simulink model "TV_2018_HIL"  (R2016a)
settings: Solver=FixedStepAuto  StartTime=0.0  StopTime=inf  FixedStep=0.001  RelTol=1e-3
PreLoadFcn:
  | TV_2017_parameters
values from neighbouring files (symbols this model uses):
  battery_voltage = single(530)    [HIL_parameters.m]    (also in HIL_parameters_2018.m; TV_2017_parameters.m; TV_2017_parameters_VD.m)
  car_params = Simulink_Car_params    [HIL_parameters.m]    (also in HIL_parameters_2018.m; TV_2017_parameters.m; TV_2017_parameters_VD.m)
  i_Diff = 16    [HIL_parameters.m]    (also in HIL_parameters_2018.m; TV_2017_parameters.m)
  Kp = 1    [HIL_parameters.m]    (also in HIL_parameters_2018.m; TV_2017_parameters.m; TV_2017_parameters_VD.m)
  motor_data = struct    [HIL_parameters.m]    (also in HIL_parameters_2018.m; TV_2017_parameters.m)
  powerLimitControl = Simulink_el    [HIL_parameters.m]    (also in HIL_parameters_2018.m; TV_2017_parameters.m; TV_2017_parameters_VD.m)
  settings = Simulink_Settings    [HIL_parameters.m]    (also in HIL_parameters_2018.m; TV_2017_parameters.m; TV_2017_parameters_VD.m)
  SpdC_BCC = 0    [HIL_parameters.m]    (also in HIL_parameters_2018.m; TV_2017_parameters.m; TV_2017_parameters_VD.m)
  Speed_Neg_sat = -21    [HIL_parameters.m]    (also in HIL_parameters_2018.m; TV_2017_parameters.m; TV_2017_parameters_VD.m)
  Speed_Pos_sat = 21    [HIL_parameters.m]    (also in HIL_parameters_2018.m; TV_2017_parameters.m; TV_2017_parameters_VD.m)
  SteeringAngleFL = [-23.80 -22.65 -21.50 -20.34 -19.18 -18.03 -16.86 -15.70 -14.53 -13.35 -12.18 -10.99 -9.80 -8.61 -7.40 -6.19 -4.97 -3.75 -2.51 -1.26 0 1.27 2.56 3.85 5.17 6.50 7.84 9.21 10.59 12.00 13.42 14.88 16.36 17.87 19.41 20.99 22.61 24.26 25.97 27.73 29.54]    [CarSetupAnalysis2018.m]    (also in HIL_parameters_2018.m; TV_2017_parameters.m; TV_2017_parameters_VD.m = [-24.129 -22.950 -21.772 -20.593 -19.413 -18.232 -17.050 -15)
  SteeringAngleFR = [-29.54 -27.73 -25.97 -24.26 -22.61 -20.99 -19.41 -17.87 -16.36 -14.88 -13.42 -12.00 -10.59 -9.21 -7.84 -6.50 -5.17 -3.85 -2.56 -1.27 0 1.26 2.51 3.75 4.97 6.19 7.40 8.61 9.80 10.99 12.18 13.35 14.53 15.70 16.86 18.03 19.18 20.34 21.50 22.65 23.80]    [CarSetupAnalysis2018.m]    (also in HIL_parameters_2018.m; TV_2017_parameters.m; TV_2017_parameters_VD.m = [-29.3050 -27.5340 -25.8140 -24.1410 -22.5110 -20.9180 -19.3)
  SteeringWhAngle = [-105 -99.75 -94.5 -89.25 -84 -78.75 -73.5 -68.25 -63 -57.75 -52.5 -47.25 -42 -36.75 -31.5 -26.25 -21.0 -15.75 -10.5 -5.25 0.0 5.25 10.50 15.75 21.00 26.25 31.50 36.75 42.00 47.25 52.50 57.75  63.00 68.25 73.50 78.75 84.00 89.25 94.50 99.75 105.00]    [TV_2017_parameters_VD.m]
  Tn_n = 0    [HIL_parameters.m]    (also in HIL_parameters_2018.m; TV_2017_parameters.m; TV_2017_parameters_VD.m)
  tractionControl = Simulink_tc    [HIL_parameters.m]    (also in HIL_parameters_2018.m; IterativeTractionControlTuning.m; TV_2017_parameters.m; TV_2017_parameters_VD.m)
  yawMomentGenerator = struct    [HIL_parameters.m]    (also in HIL_parameters_2018.m = Simulink_yawRate2; TV_2017_parameters.m = Simulink_yawRate2)
  yawRateControl = Simulink_yawRate    [HIL_parameters.m]    (also in HIL_parameters_2018.m; TV_2017_parameters.m; TV_2017_parameters_VD.m)
undefined symbols (not defined in the file or in its folder): canChannel, DiscIntNeverNeededParam, magnitude, speedEstimation, TC_Decr_Gas, TC_Derivative, TC_Incr_Gas, TC_On, TC_Relay_Off, TC_Relay_On
libraries: CarMaker4SL x366, simulink_extras x63, canmsglib x55, canlib x41, simulink x37, dspfdesign x2, sldrtlib x1
(part 4 of 15)

== system TV_2018_HIL/CarMaker/Send sensor data and driver input to microcontroller /If Action Subsystem1 ==
  Action Port : ActionPort
  CAN Pack24 : canmsglib/CAN Pack  MsgList=(none)  MsgName=CAN Msg  MsgIDType=Standard (11-bit identifier)  MsgIdentifier=DRIVE_ENABLE  MsgLength=0  NSignals=0  StartBits=0  SignalSizes=0  ByteOrders=0  DataTypes=0  MultiplexTypes=0  MultiplexValues=0  Factors=0  Offsets=0  Minimums=0  Maximums=0  Remote=off
      settings: DataFormat=manually specified signals
  CAN Transmit24 : canlib/CAN Transmit  BlockHandle=3115.0001  DeviceMenu=(none)  Device=PEAK-System PCAN-PCI Express (PCAN_PCIBUS1)  ObjConstructor=canChannel('PEAK-System', 'PCAN_PCIBUS1')  EnablePeriodicTransmit=off  MessagePeriod=1.000

== system TV_2018_HIL/CarMaker/Send sensor data and driver input to microcontroller /If Action Subsystem2 ==
  Action Port : ActionPort  ActionType=case
  CAN Pack23 : canmsglib/CAN Pack  MsgList=(none)  MsgName=CAN Msg  MsgIDType=Standard (11-bit identifier)  MsgIdentifier=RESET_INVERTER  MsgLength=0  NSignals=0  StartBits=0  SignalSizes=0  ByteOrders=0  DataTypes=0  MultiplexTypes=0  MultiplexValues=0  Factors=0  Offsets=0  Minimums=0  Maximums=0  Remote=off
      settings: DataFormat=manually specified signals
  CAN Transmit23 : canlib/CAN Transmit  BlockHandle=3119.0001  DeviceMenu=(none)  Device=PEAK-System PCAN-PCI Express (PCAN_PCIBUS1)  ObjConstructor=canChannel('PEAK-System', 'PCAN_PCIBUS1')  EnablePeriodicTransmit=off  MessagePeriod=1.000
  wires:
  CAN Pack23/1 -> CAN Transmit23/1

== system TV_2018_HIL/CarMaker/Send sensor data and driver input to microcontroller /Push Button ==

== system TV_2018_HIL/CarMaker/Send sensor data and driver input to microcontroller /Push Button1 ==

== system TV_2018_HIL/CarMaker/Send sensor data and driver input to microcontroller /Push Button2 ==

== system TV_2018_HIL/CarMaker/Send sensor data and driver input to microcontroller /Trash ==
  In1 : Inport
  In2 : Inport  Port=2
  In3 : Inport  Port=3
  In4 : Inport  Port=4
  In5 : Inport  Port=5
  In6 : Inport  Port=6
  In7 : Inport  Port=7
  In8 : Inport  Port=8
  In9 : Inport  Port=9
  In10 : Inport  Port=10
  In11 : Inport  Port=11
  In12 : Inport  Port=12
  In13 : Inport  Port=13
  In14 : Inport  Port=14
  In15 : Inport  Port=15
  In16 : Inport  Port=16
  In17 : Inport  Port=17
  In18 : Inport  Port=18
  CAN Pack : canmsglib/CAN Pack  Commented=on  MsgList=(none)  MsgName=CAN Msg  MsgIDType=Standard (11-bit identifier)  MsgIdentifier=ACD_DAMPER_FL_ID  MsgLength=2  SignalInfo=FL$0$16$1$1$1$0$1$0$-Inf$Inf$#  NSignals=1  StartBits=str2num('[int32(0)]')  SignalSizes=str2num('[int32(16)]')  ByteOrders=str2num('[int32(1)]')  DataTypes=str2num('[int32(1)]')  MultiplexTypes=str2num('[int32(1)]')  MultiplexValues=str2num('[double(0)]')  Factors=str2num('[double(1)]')  Offsets=str2num('[double(0)]')  Minimums=str2num('[double(-Inf)]')  Maximums=str2num('[double(Inf)]')  Remote=off
      settings: DataFormat=manually specified signals
  CAN Pack1 : canmsglib/CAN Pack  Commented=on  MsgList=(none)  MsgName=CAN Msg  MsgIDType=Standard (11-bit identifier)  MsgIdentifier=ACD_DAMPER_FR_ID  MsgLength=8  NSignals=0  StartBits=0  SignalSizes=0  ByteOrders=0  DataTypes=0  MultiplexTypes=0  MultiplexValues=0  Factors=0  Offsets=0  Minimums=0  Maximums=0  Remote=off
      settings: DataFormat=manually specified signals
  CAN Pack12 : canmsglib/CAN Pack  Commented=on  MsgList=(none)  MsgName=RPM  MsgIDType=Standard (11-bit identifier)  MsgIdentifier=502  MsgLength=8  SignalInfo=RPM_FL$0$16$1$1$1$0$1$0$-Inf$Inf$#RPM_FR$16$16$1$1$1$0$1$0$-Inf$Inf$#RPM_RL$32$16$1$1$1$0$1$0$-Inf$Inf$#RPM_RR$48$16$1$1$1$0$1$0$-Inf$Inf$#  NSignals=4  StartBits=str2num('[int32(0);int32(16);int32(32);int32(48)]')  SignalSizes=str2num('[int32(16);int32(16);int32(16);int32(16)]')  ByteOrders=str2num('[int32(1);int32(1);int32(1);int32(1)]')  DataTypes=str2num('[int32(1);int32(1);int32(1);int32(1)]')  MultiplexTypes=str2num('[int32(1);int32(1);int32(1);int32(1)]')  MultiplexValues=str2num('[double(0);double(0);double(0);double(0)]')  Factors=str2num('[double(1);double(1);double(1);double(1)]')  Offsets=str2num('[double(0);double(0);double(0);double(0)]')  Minimums=str2num('[double(-Inf);double(-Inf);double(-Inf);double(-Inf)]')  Maximums=str2num('[double(Inf);double(Inf);double(Inf);double(Inf)]')  Remote=off
      settings: DataFormat=manually specified signals
  CAN Pack2 : canmsglib/CAN Pack  Commented=on  MsgList=(none)  MsgName=CAN Msg  MsgIDType=Standard (11-bit identifier)  MsgIdentifier=ACD_DAMPER_RL_ID  MsgLength=8  NSignals=0  StartBits=0  SignalSizes=0  ByteOrders=0  DataTypes=0  MultiplexTypes=0  MultiplexValues=0  Factors=0  Offsets=0  Minimums=0  Maximums=0  Remote=off
      settings: DataFormat=manually specified signals
  CAN Pack20 : canmsglib/CAN Pack  Commented=on  MsgList=(none)  MsgName=Fz  MsgIDType=Standard (11-bit identifier)  MsgIdentifier=500  MsgLength=8  SignalInfo=Fz_FL$0$16$1$2$1$0$1$0$-Inf$Inf$#Fz_FR$16$16$1$2$1$0$1$0$-Inf$Inf$#Fz_RL$32$16$1$2$1$0$1$0$-Inf$Inf$#Fz_RR$48$16$1$2$1$0$1$0$-Inf$Inf$#  NSignals=4  StartBits=str2num('[int32(0);int32(16);int32(32);int32(48)]')  SignalSizes=str2num('[int32(16);int32(16);int32(16);int32(16)]')  ByteOrders=str2num('[int32(1);int32(1);int32(1);int32(1)]')  DataTypes=str2num('[int32(2);int32(2);int32(2);int32(2)]')  MultiplexTypes=str2num('[int32(1);int32(1);int32(1);int32(1)]')  MultiplexValues=str2num('[double(0);double(0);double(0);double(0)]')  Factors=str2num('[double(1);double(1);double(1);double(1)]')  Offsets=str2num('[double(0);double(0);double(0);double(0)]')  Minimums=str2num('[double(-Inf);double(-Inf);double(-Inf);double(-Inf)]')  Maximums=str2num('[double(Inf);double(Inf);double(Inf);double(Inf)]')  Remote=off
      settings: DataFormat=manually specified signals
  CAN Pack3 : canmsglib/CAN Pack  Commented=on  MsgList=(none)  MsgName=CAN Msg  MsgIDType=Standard (11-bit identifier)  MsgIdentifier=ACD_DAMPER_RR_ID  MsgLength=8  NSignals=0  StartBits=0  SignalSizes=0  ByteOrders=0  DataTypes=0  MultiplexTypes=0  MultiplexValues=0  Factors=0  Offsets=0  Minimums=0  Maximums=0  Remote=off
      settings: DataFormat=manually specified signals
  CAN Pack6 : canmsglib/CAN Pack  Commented=on  MsgList=(none)  MsgName=Senors  MsgIDType=Standard (11-bit identifier)  MsgIdentifier=501  MsgLength=8  SignalInfo=gas$0$8$1$2$1$0$1$0$-Inf$Inf$#kers$8$8$1$2$1$0$1$0$-Inf$Inf$#steering$16$16$1$1$1$0$1$0$-Inf$Inf$#vx$32$16$1$1$1$0$1$0$-Inf$Inf$#yawrate$48$16$1$1$1$0$1$0$-Inf$Inf$#  NSignals=5  StartBits=str2num('[int32(0);int32(8);int32(16);int32(32);int32(48)]')  SignalSizes=str2num('[int32(8);int32(8);int32(16);int32(16);int32(16)]')  ByteOrders=str2num('[int32(1);int32(1);int32(1);int32(1);int32(1)]')  DataTypes=str2num('[int32(2);int32(2);int32(1);int32(1);int32(1)]')  MultiplexTypes=str2num('[int32(1);int32(1);int32(1);int32(1);int32(1)]')  MultiplexValues=str2num('[double(0);double(0);double(0);double(0);double(0)]')  Factors=str2num('[double(1);double(1);double(1);double(1);double(1)]')  Offsets=str2num('[double(0);double(0);double(0);double(0);double(0)]')  Minimums=str2num('[double(-Inf);double(-Inf);double(-Inf);double(-Inf);double(-Inf)]')  Maximums=str2num('[double(Inf);double(Inf);double(Inf);double(Inf);double(Inf)]')  Remote=off
      settings: DataFormat=manually specified signals
  CAN Pack8 : canmsglib/CAN Pack  Commented=on  MsgList=(none)  MsgName=CAN Msg  MsgIDType=Standard (11-bit identifier)  MsgIdentifier=2  MsgLength=8  SignalInfo=Signal1$0$8$1$1$1$0$1$0$-Inf$Inf$#  NSignals=1  StartBits=str2num('[int32(0)]')  SignalSizes=str2num('[int32(8)]')  ByteOrders=str2num('[int32(1)]')  DataTypes=str2num('[int32(1)]')  MultiplexTypes=str2num('[int32(1)]')  MultiplexValues=str2num('[double(0)]')  Factors=str2num('[double(1)]')  Offsets=str2num('[double(0)]')  Minimums=str2num('[double(-Inf)]')  Maximums=str2num('[double(Inf)]')  Remote=off
      settings: DataFormat=manually specified signals
  CAN Transmit : canlib/CAN Transmit  Commented=on  BlockHandle=19242.0006  DeviceMenu=Kvaser Virtual 1 (Channel 1)  Device=PEAK-System PCAN-PCI Express (PCAN_PCIBUS1)  ObjConstructor=CANTRANCONSTRUCTOR  EnablePeriodicTransmit=off  MessagePeriod=1.000
  CAN Transmit1 : canlib/CAN Transmit  Commented=on  BlockHandle=19243.0006  DeviceMenu=Kvaser Virtual 1 (Channel 1)  Device=PEAK-System PCAN-USB (PCAN_USBBUS1)  ObjConstructor=canChannel('PEAK-System', 'PCAN_USBBUS1')  EnablePeriodicTransmit=on  MessagePeriod=0.01
  CAN Transmit15 : canlib/CAN Transmit  Commented=on  BlockHandle=19244.0006  DeviceMenu=Kvaser Virtual 1 (Channel 1)  Device=PEAK-System PCAN-USB (PCAN_USBBUS1)  ObjConstructor=canChannel('PEAK-System', 'PCAN_USBBUS1')  EnablePeriodicTransmit=on  MessagePeriod=0.01
  CAN Transmit19 : canlib/CAN Transmit  Commented=on  BlockHandle=19245.0006  DeviceMenu=Kvaser Virtual 1 (Channel 1)  Device=PEAK-System PCAN-USB (PCAN_USBBUS1)  ObjConstructor=canChannel('PEAK-System', 'PCAN_USBBUS1')  EnablePeriodicTransmit=on  MessagePeriod=0.01
  CAN Transmit2 : canlib/CAN Transmit  Commented=on  BlockHandle=19246.0006  DeviceMenu=Kvaser Virtual 1 (Channel 1)  Device=PEAK-System PCAN-PCI Express (PCAN_PCIBUS1)  ObjConstructor=CANTRANCONSTRUCTOR  EnablePeriodicTransmit=off  MessagePeriod=1.000
  CAN Transmit3 : canlib/CAN Transmit  Commented=on  BlockHandle=19247.0006  DeviceMenu=Kvaser Virtual 1 (Channel 1)  Device=PEAK-System PCAN-PCI Express (PCAN_PCIBUS1)  ObjConstructor=CANTRANCONSTRUCTOR  EnablePeriodicTransmit=off  MessagePeriod=1.000
  CAN Transmit4 : canlib/CAN Transmit  Commented=on  BlockHandle=19248.0006  DeviceMenu=Kvaser Virtual 1 (Channel 1)  Device=PEAK-System PCAN-PCI Express (PCAN_PCIBUS1)  ObjConstructor=CANTRANCONSTRUCTOR  EnablePeriodicTransmit=off  MessagePeriod=1.000
  CAN Transmit8 : canlib/CAN Transmit  Commented=on  BlockHandle=19249.0006  DeviceMenu=Kvaser Virtual 1 (Channel 1)  Device=PEAK-System PCAN-PCI Express (PCAN_PCIBUS1)  ObjConstructor=canChannel('PEAK-System', 'PCAN_PCIBUS1')  EnablePeriodicTransmit=off  MessagePeriod=1.000
  Constant5 : Constant  Commented=on
  Constant6 : Constant  Commented=on
  Scope11 : Scope  Commented=on
  Out1 : Outport
  wires:
  CAN Pack8/1 -> CAN Transmit8/1
  In9/1 -> CAN Pack6/2
  In8/1 -> CAN Pack6/1
  In10/1 -> CAN Pack6/3
  In18/1 -> Scope11/1
  In3/1 -> CAN Pack3/1
  In15/1 -> CAN Transmit15/1
  CAN Pack12/1 -> Out1/1
  In17/1 -> CAN Pack12/4
  In4/1 -> CAN Pack20/1
  In5/1 -> CAN Pack20/2
  In14/1 -> CAN Pack12/2
  In7/1 -> CAN Pack20/4
  In12/1 -> CAN Pack6/5
  In2/1 -> CAN Pack2/1
  In13/1 -> CAN Pack12/1
  In16/1 -> CAN Pack12/3
  In11/1 -> CAN Pack6/4
  In1/1 -> CAN Pack1/1
  In6/1 -> CAN Pack20/3
  CAN Pack6/1 -> CAN Transmit1/1
  CAN Pack3/1 -> CAN Transmit4/1
  CAN Pack/1 -> CAN Transmit/1
  Constant5/1 -> CAN Pack/1
  CAN Pack1/1 -> CAN Transmit2/1
  CAN Pack20/1 -> CAN Transmit19/1
  CAN Pack2/1 -> CAN Transmit3/1
  Constant6/1 -> CAN Pack8/1

== system TV_2018_HIL/CarMaker/Send sensor data and driver input to microcontroller /force2 0.1mmDamperFront ==
  In1 : Inport
  Constant2 : Constant  Value=800
  Gain : Gain  Gain=1/car_params.spring_constant_front
  Sum : Sum  Inputs=|++
  sensor scale : Gain  Gain=1/0.1
  Out1 : Outport
  wires:
  Constant2/1 -> Sum/2
  In1/1 -> Sum/1
  Sum/1 -> Gain/1
  Gain/1 -> sensor scale/1
  sensor scale/1 -> Out1/1

== system TV_2018_HIL/CarMaker/Send sensor data and driver input to microcontroller /force2mmDamperFront1 ==
  In1 : Inport
  Constant2 : Constant  Value=800
  Gain1 : Gain  Gain=1/car_params.spring_constant_front
  Sum : Sum  Inputs=|++
  sensor scale : Gain  Gain=1/0.1
  Out1 : Outport
  wires:
  Constant2/1 -> Sum/2
  In1/1 -> Sum/1
  Sum/1 -> Gain1/1
  Gain1/1 -> sensor scale/1
  sensor scale/1 -> Out1/1

== system TV_2018_HIL/CarMaker/Send sensor data and driver input to microcontroller /force2mmDamperRear ==
  In1 : Inport
  Constant2 : Constant  Value=1600
  Gain : Gain  Gain=1/car_params.spring_constant_rear
  Sum : Sum  Inputs=|++
  sensor scale : Gain  Gain=1/0.1
  Out1 : Outport
  wires:
  Constant2/1 -> Sum/2
  In1/1 -> Sum/1
  Sum/1 -> Gain/1
  Gain/1 -> sensor scale/1
  sensor scale/1 -> Out1/1

== system TV_2018_HIL/CarMaker/Send sensor data and driver input to microcontroller /force2mmDamperRear1 ==
  In1 : Inport
  Constant2 : Constant  Value=1600
  Gain : Gain  Gain=1/car_params.spring_constant_rear
  Sum : Sum  Inputs=|++
  sensor scale : Gain  Gain=1/0.1
  Out1 : Outport
  wires:
  Constant2/1 -> Sum/2
  In1/1 -> Sum/1
  Sum/1 -> Gain/1
  Gain/1 -> sensor scale/1
  sensor scale/1 -> Out1/1

== system TV_2018_HIL/CarMaker/Subsystem/Control Output to CarMaker model  ==
  "Ti_pos " : Inport
  Ti_neg : Inport  Port=2
  wi_ref : Inport  Port=3
  Bus Selector : BusSelector  OutputSignals=FL,FR,RL,RR
  Bus Selector1 : BusSelector  OutputSignals=FL,FR,RL,RR
  Bus Selector2 : BusSelector  OutputSignals=FL,FR,RL,RR
  Data Type Conversion{,1..11} (12 alike) : DataTypeConversion  OutDataTypeStr=double
  Gain{,1..7} (8 alike) : Gain  Gain=car_params.Mn
  Scope4 : Scope
  Ti_To_CarMaker : Scope  NumInputPorts=4
  Write CM Dict : CarMaker4SL/Write CM Dict  xname=T_req_RR  xsync=off
  Write CM Dict1 : CarMaker4SL/Write CM Dict  xname=T_req_RL  xsync=off
  Write CM Dict10 : CarMaker4SL/Write CM Dict  xname=Tlim_pos_RL  xsync=off
  Write CM Dict11 : CarMaker4SL/Write CM Dict  xname=Tlim_pos_RR  xsync=off
  Write CM Dict16 : CarMaker4SL/Write CM Dict  xname=Tlim_neg_FL  xsync=off
  Write CM Dict17 : CarMaker4SL/Write CM Dict  xname=Tlim_neg_FR  xsync=off
  Write CM Dict18 : CarMaker4SL/Write CM Dict  xname=Tlim_neg_RL  xsync=off
  Write CM Dict19 : CarMaker4SL/Write CM Dict  xname=Tlim_neg_RR  xsync=off
  Write CM Dict2 : CarMaker4SL/Write CM Dict  xname=T_req_FR  xsync=off
  Write CM Dict3 : CarMaker4SL/Write CM Dict  xname=T_req_FL  xsync=off
  Write CM Dict4 : CarMaker4SL/Write CM Dict  xname=w_set_FR  xsync=off
  Write CM Dict5 : CarMaker4SL/Write CM Dict  xname=w_set_RL  xsync=off
  Write CM Dict6 : CarMaker4SL/Write CM Dict  xname=w_set_RR  xsync=off
  Write CM Dict7 : CarMaker4SL/Write CM Dict  xname=Tlim_pos_FL  xsync=off
  Write CM Dict8 : CarMaker4SL/Write CM Dict  xname=w_set_FL  xsync=off
  Write CM Dict9 : CarMaker4SL/Write CM Dict  xname=Tlim_pos_FR  xsync=off
  wires:
  "Ti_pos "/1 -> Bus Selector/1
  Bus Selector/1 -> Data Type Conversion/1  "<FL>"
  Bus Selector/2 -> Data Type Conversion1/1  "<FR>"
  Bus Selector/3 -> Data Type Conversion2/1  "<RL>"
  Bus Selector/4 -> Data Type Conversion3/1  "<RR>"
  Data Type Conversion3/1 -> Gain3/1
  Bus Selector1/1 -> Data Type Conversion4/1  "<FL>"
  Bus Selector1/2 -> Data Type Conversion5/1  "<FR>"
  Bus Selector1/3 -> Data Type Conversion6/1  "<RL>"
  Bus Selector1/4 -> Data Type Conversion7/1  "<RR>"
  wi_ref/1 -> Bus Selector1/1
  Data Type Conversion4/1 -> Write CM Dict8/1
  Data Type Conversion5/1 -> Write CM Dict4/1
  Data Type Conversion6/1 -> Write CM Dict5/1
  Data Type Conversion7/1 -> Scope4/1, Write CM Dict6/1
  Data Type Conversion1/1 -> Gain1/1
  Data Type Conversion/1 -> Gain/1
  Data Type Conversion2/1 -> Gain2/1
  Ti_neg/1 -> Bus Selector2/1
  Bus Selector2/1 -> Data Type Conversion8/1  "<FL>"
  Bus Selector2/2 -> Data Type Conversion9/1  "<FR>"
  Bus Selector2/3 -> Data Type Conversion10/1  "<RL>"
  Bus Selector2/4 -> Data Type Conversion11/1  "<RR>"
  Data Type Conversion8/1 -> Gain4/1
  Data Type Conversion9/1 -> Gain5/1
  Data Type Conversion10/1 -> Gain6/1
  Data Type Conversion11/1 -> Gain7/1
  Gain/1 -> Write CM Dict3/1, Ti_To_CarMaker/1, Write CM Dict7/1
  Gain1/1 -> Ti_To_CarMaker/2, Write CM Dict9/1, Write CM Dict2/1
  Gain2/1 -> Ti_To_CarMaker/3, Write CM Dict10/1, Write CM Dict1/1
  Gain3/1 -> Ti_To_CarMaker/4, Write CM Dict11/1, Write CM Dict/1
  Gain4/1 -> Write CM Dict16/1
  Gain5/1 -> Write CM Dict17/1
  Gain6/1 -> Write CM Dict18/1
  Gain7/1 -> Write CM Dict19/1

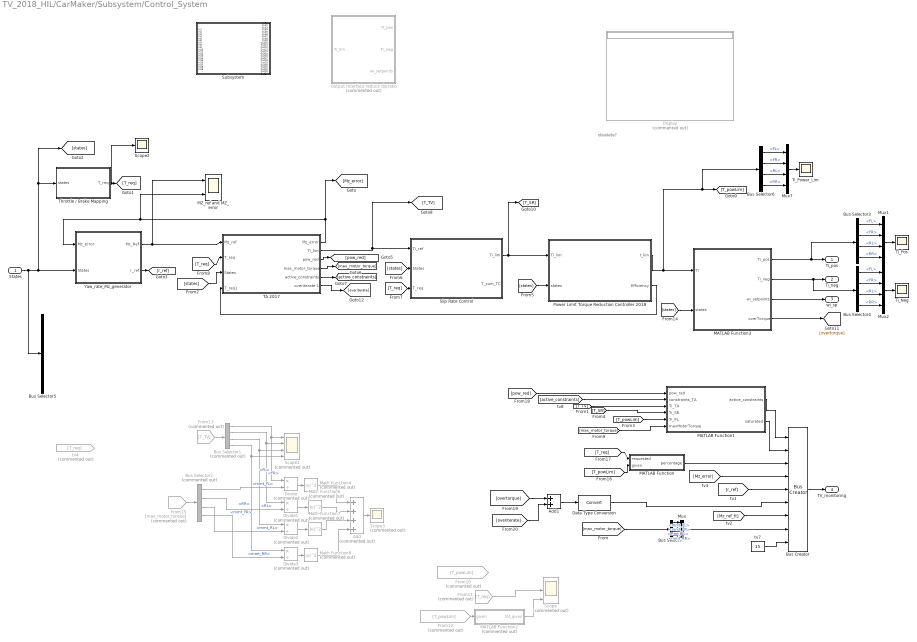
== system TV_2018_HIL/CarMaker/Subsystem/Control_System  ==
  note: obsolete?
  "States " : Inport
  Add : Sum  Commented=on  Inputs=++++
  Add1 : Sum
  Bus Creator : BusCreator  Inputs=9  OutDataTypeStr=Bus: TV_monitoring
      settings: InheritFromInputs=off
  Bus Selector : BusSelector  OutputSignals=mmt_FL,mmt_FR,mmt_RL,mmt_RR
  Bus Selector1 : BusSelector  Commented=on  OutputSignals=FL,FR,RL,RR
  Bus Selector2 : BusSelector  Commented=on  OutputSignals=mmt_FL,mmt_FR,mmt_RL,mmt_RR
  Bus Selector3 : BusSelector  OutputSignals=FL,FR,RL,RR
  Bus Selector4 : BusSelector  OutputSignals=FL,FR,RL,RR
  Bus Selector5 : BusSelector  OutputSignals=ax
  Bus Selector6 : BusSelector  OutputSignals=FL,FR,RL,RR
  Data Type Conversion : DataTypeConversion
  Display : Display  Commented=on
  Divide{,1..3} (4 alike) : Product  Commented=on  Inputs=*/
  From10 : From  Commented=on  GotoTag=T_powLim
  From11 : From  Commented=on  GotoTag=T_req
  From12 : From  Commented=on  GotoTag=T_powLim
  From13 : From  Commented=on  GotoTag=T_TV
  From15 : From  Commented=on  GotoTag=max_motor_torque
  MATLAB Function : MATLAB Function  TreatAsAtomicUnit=on
  MATLAB Function1 : MATLAB Function  TreatAsAtomicUnit=on
  MATLAB Function2 : MATLAB Function  Commented=on  TreatAsAtomicUnit=on
  MATLAB Function3 : MATLAB Function  TreatAsAtomicUnit=on
  MZ_ref and MZ_error : Scope  NumInputPorts=2
  Math Function{4,6..8} (4 alike) : Math  Commented=on  Operator=magnitude^2  SaturateOnIntegerOverflow=on
  Mux{,1..2,7} (4 alike) : Mux
  Output Interface reduce slipratio : Subsystem  Commented=on
  Power Limit Torque Reduction Controller 2018 : Subsystem
  Scope : Scope  Commented=on  NumInputPorts=3
  Scope1 : Scope  Commented=on  NumInputPorts=4
  Scope2 : Scope
  Scope3 : Scope  Commented=on
  "Slip Rate Control " : Subsystem
  Subsystem : Subsystem
  TA 2017 : Subsystem
  Throttle / Brake Mapping : MATLAB Function  TreatAsAtomicUnit=on
  Ti_Neg : Scope
  Ti_Pos : Scope
  Ti_Power_Lim : Scope
  Yaw_rate_Mz_generator : Subsystem
  tv4 : From  Commented=on  GotoTag=T_req
  tv7 : Constant  Value=15  OutDataTypeStr=single
  "Ti_pos " : Outport
  Ti_neg : Outport  Port=2
  wi_sp : Outport  Port=3
  TV_monitoring : Outport  Port=4
  wires:
  Throttle / Brake Mapping/1(T_req) -> Scope2/1, [T_req]
  TA 2017/1("Mz_error ") -> [Mz_error], MZ_ref and MZ_error/2, Yaw_rate_Mz_generator/1(Mz_error)
  [states] -> TA 2017/3("States ")
  TA 2017/2(Ti_lim) -> "Slip Rate Control "/1(Ti_ref), [T_TV]
  [states] -> Power Limit Torque Reduction Controller 2018/2(states)
  [T_req] -> TA 2017/2(T_req)
  "States "/1 -> Bus Selector5/1, [states], Throttle / Brake Mapping/1(states), Yaw_rate_Mz_generator/2(States)
  Bus Creator/1 -> TV_monitoring/1
  TA 2017/3(pow_red) -> [pow_red]
  [active_constraints] -> MATLAB Function1/2(constraints_TA)
  TA 2017/4(max_motor_torque) -> [max_motor_torque]
  TA 2017/5(active_constraints) -> [active_constraints]
  [pow_red] -> MATLAB Function1/1(pow_red)
  [T_powLim] -> MATLAB Function/2(given)
  [T_req] -> MATLAB Function/1(requested)
  [Mz_error] -> Bus Creator/4
  MATLAB Function/1(percentage) -> Bus Creator/3
  tv7/1 -> Bus Creator/9
  [max_motor_torque] -> Bus Selector/1
  [Mz_ref_tt] -> Bus Creator/7
  [r_ref] -> Bus Creator/5
  Add1/1 -> Data Type Conversion/1
  MATLAB Function3/3(wi_setpoints) -> wi_sp/1
  MATLAB Function3/1(Ti_pos) -> Bus Selector3/1, "Ti_pos "/1
  MATLAB Function3/2(Ti_neg) -> Bus Selector4/1, Ti_neg/1
  Mux/1 -> Bus Creator/8
  Bus Selector/1 -> Mux/1  "<mmt_FL>"
  Bus Selector/2 -> Mux/2  "<mmt_FR>"
  Bus Selector/3 -> Mux/3  "<mmt_RL>"
  Bus Selector/4 -> Mux/4  "<mmt_RR>"
  [states] -> "Slip Rate Control "/2("States ")
  [T_req] -> "Slip Rate Control "/3(T_req)
  "Slip Rate Control "/1(Ti_lim) -> [T_SR], Power Limit Torque Reduction Controller 2018/1(Ti_lim)
  [T_TV] -> MATLAB Function1/3(Ti_TA)
  [T_powLim] -> MATLAB Function1/5(Ti_PL)
  [T_SR] -> MATLAB Function1/4(Ti_SR)
  [max_motor_torque] -> MATLAB Function1/6(maxMotorTorque)
  MATLAB Function1/2(saturated) -> Bus Creator/2
  From11/1 -> Scope/2
  From12/1 -> MATLAB Function2/1(given)
  MATLAB Function2/1(tot_given) -> Scope/3
  From13/1 -> Bus Selector1/1
  Bus Selector1/1 -> Divide/1, Scope1/1  "<FL>"
  Bus Selector1/2 -> Divide1/1, Scope1/2  "<FR>"
  Bus Selector1/3 -> Divide2/1, Scope1/3  "<RL>"
  Bus Selector1/4 -> Divide3/1, Scope1/4  "<RR>"
  MATLAB Function1/1(active_constraints) -> Bus Creator/1
  Bus Selector2/1 -> Divide/2  "<mmt_FL>"
  Bus Selector2/2 -> Divide1/2  "<mmt_FR>"
  Bus Selector2/3 -> Divide2/2  "<mmt_RL>"
  Bus Selector2/4 -> Divide3/2  "<mmt_RR>"
  From15/1 -> Bus Selector2/1
  Divide/1 -> Math Function4/1
  Divide1/1 -> Math Function6/1
  Divide2/1 -> Math Function7/1
  Divide3/1 -> Math Function8/1
  Math Function4/1 -> Add/1
  Math Function6/1 -> Add/2
  Math Function7/1 -> Add/3
  Math Function8/1 -> Add/4
  Add/1 -> Scope3/1
  [states] -> MATLAB Function3/2(states)
  Power Limit Torque Reduction Controller 2018/1(t_lim) -> Bus Selector6/1, [T_powLim], MATLAB Function3/1(Ti)
  MATLAB Function3/4(overTorque) -> [overtorque]
  TA 2017/6(overiterate 1) -> [overiterate]
  [overtorque] -> Add1/1
  [overiterate] -> Add1/2
  Data Type Conversion/1 -> Bus Creator/6
  Bus Selector6/1 -> Mux7/1  "<FL>"
  Bus Selector6/2 -> Mux7/2  "<FR>"
  Bus Selector6/3 -> Mux7/3  "<RL>"
  Bus Selector6/4 -> Mux7/4  "<RR>"
  Mux7/1 -> Ti_Power_Lim/1
  Bus Selector3/1 -> Mux1/1  "<FL>"
  Bus Selector3/2 -> Mux1/2  "<FR>"
  Bus Selector3/3 -> Mux1/3  "<RL>"
  Bus Selector3/4 -> Mux1/4  "<RR>"
  Mux1/1 -> Ti_Pos/1
  Bus Selector4/1 -> Mux2/1  "<FL>"
  Bus Selector4/2 -> Mux2/2  "<FR>"
  Bus Selector4/3 -> Mux2/3  "<RL>"
  Bus Selector4/4 -> Mux2/4  "<RR>"
  Mux2/1 -> Ti_Neg/1
  Yaw_rate_Mz_generator/1(Mz_Ref) -> MZ_ref and MZ_error/1, TA 2017/1(Mz_ref)
  Yaw_rate_Mz_generator/2(r_ref) -> [r_ref]
  Power Limit Torque Reduction Controller 2018/2(Efficiency) -> TA 2017/4(T_req1)

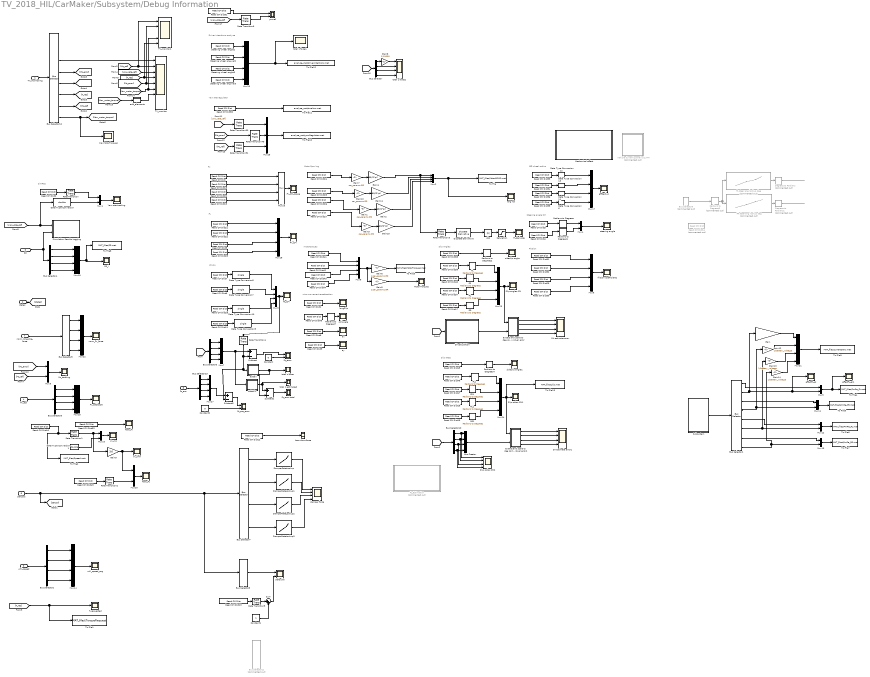
== system TV_2018_HIL/CarMaker/Subsystem/Debug Information  ==
  note: SimRes
  note: Eff wheel radius
  note: motortorques
  note: Friction
  note: FZ CM
  note: Fy
  note: FX
  note: misc movement acceleration
  note: Steering angle CM
  note: Motor Rpm log
  note: Slip Angles
  note: Slip rates
  note: Yaw rate regulator
  note: Driver intentions analyze
  TV_monitoring : Inport
  states : Inport  Port=2
  whl_speed : Inport  Port=3
  Fx_est : Inport  Port=4
  "SR " : Inport  Port=5
  Sensors : Inport  Port=6
  norm_long_tire_force : Inport  Port=7
  Fz_acc : Inport  Port=8
  Abs : Abs
  "Aero downforce " : Scope
  Aero_Fx : Scope
  Aero_Fz : Scope
  Bus Creator : BusCreator  Inputs=4
  Bus Selector : BusSelector  OutputSignals=power,Input_throttle,Input_brake,KERS_pos
  Bus Selector1 : BusSelector  OutputSignals=Pm_FL,Pe_FL,Pm_FR,Pe_FR,Pm_RL,Pe_RL,Pm_RR,Pe_RR
  Bus Selector10 : BusSelector  OutputSignals=SR_FL,SR_FR,SR_RL,SR_RR
  Bus Selector11 : BusSelector  Commented=on  OutputSignals=steering_wheel_angle
  Bus Selector12 : BusSelector  OutputSignals=active_contraints,saturated_constraints,percentage_delivered_torque,Mz_error,yaw_rate_ref,T_req,Mz_ref,maxMotorTorque
  Bus Selector{2..5,13} (5 alike) : BusSelector  OutputSignals=FL,FR,RL,RR
  Bus Selector6 : BusSelector  OutputSignals=Fz_FL,Fz_FR,Fz_RL,Fz_RR
  Bus Selector7 : BusSelector  OutputSignals=damper_rate_FL,damper_rate_FR,damper_rate_RL,damper_rate_RR
  Bus Selector8 : BusSelector  OutputSignals=steering_wheel_angle
  Bus Selector9 : BusSelector  Commented=on  OutputSignals=steering_wheel_angle
  Constant : Constant  Value=0
  Constant1 : Constant
  Constant2 : Constant  Value=0
  DamperRateLookup : Lookup_n-D  NumberOfTableDimensions=1  BreakpointsForDimension1=car_params.damper_table_breakpoint;  Table=car_params.damper_pull_push_values_front;  ExtrapMethod=Clip  UseLastTableValue=on  InternalRulePriority=Speed  RndMeth=Simplest  InputSameDT=on
  DamperRateLookup1 : Lookup_n-D  NumberOfTableDimensions=1  BreakpointsForDimension1=car_params.damper_table_breakpoint;  Table=car_params.damper_pull_push_values_front;  ExtrapMethod=Clip  UseLastTableValue=on  InternalRulePriority=Speed  RndMeth=Simplest  InputSameDT=on
  DamperRateLookup2 : Lookup_n-D  NumberOfTableDimensions=1  BreakpointsForDimension1=car_params.damper_table_breakpoint;  Table=car_params.damper_pull_push_values_rear;  ExtrapMethod=Clip  UseLastTableValue=on  InternalRulePriority=Speed  RndMeth=Simplest  InputSameDT=on
  DamperRateLookup3 : Lookup_n-D  NumberOfTableDimensions=1  BreakpointsForDimension1=car_params.damper_table_breakpoint;  Table=car_params.damper_pull_push_values_rear;  ExtrapMethod=Clip  UseLastTableValue=on  InternalRulePriority=Speed  RndMeth=Simplest  InputSameDT=on
  Data Type Conversion : DataTypeConversion  OutDataTypeStr=double
  Data Type Conversion1 : DataTypeConversion  OutDataTypeStr=double
  Data Type Conversion{6..13} (8 alike) : DataTypeConversion  OutDataTypeStr=single
  Degrees to Radians : simulink_extras/Transformations/Degrees to Radians  Commented=on
  Degrees to Radians1 : simulink_extras/Transformations/Degrees to Radians  Commented=on
  Discrete Derivative : simulink/Discrete/Discrete Derivative  gainval=1.0  ICPrevScaledInput=0.0  InputProcessing=Inherited  OutMin=[]  OutMax=[]  OutDataType=fixdt(1, 16)  OutScaling=2^-10  DoSatur=off
  Extract and scale to deg compare to CM output in individual error : Subsystem
  Extract and scale to deg compare to CM output in individual error1 : Subsystem
  FL : simulink_extras/Transformations/Radians to Degrees
  FL steer ang lookup deg : Lookup_n-D  Commented=on  NumberOfTableDimensions=1  BreakpointsForDimension1=SteeringWhAngle  Table=SteeringAngleFL  ExtrapMethod=Clip  UseLastTableValue=on  InternalRulePriority=Speed  RndMeth=Simplest  InputSameDT=on
  FL1 : simulink_extras/Transformations/Radians to Degrees
  FR : simulink_extras/Transformations/Radians to Degrees
  FR steer ang lookup deg : Lookup_n-D  Commented=on  NumberOfTableDimensions=1  BreakpointsForDimension1=SteeringWhAngle  Table=SteeringAngleFR  ExtrapMethod=Clip  UseLastTableValue=on  InternalRulePriority=Speed  RndMeth=Simplest  InputSameDT=on
  FR1 : simulink_extras/Transformations/Radians to Degrees
  FY_CM : Scope
  Fl_derivate : Scope
  Fx_CM_scope : Scope
  Fx_estScope : Scope
  Fz_CM : Scope
  Fz_Estimation : Subsystem  Commented=on  TreatAsAtomicUnit=on
  Fz_acc_error : Scope  NumInputPorts=2
  Fz_error : Scope  NumInputPorts=2
  Fz_error total : Scope
  Gain{,12..14} (4 alike) : Gain  Gain=1/battery_voltage
  Gain{1,3,7,10} (4 alike) : Gain  Gain=car_params.GR
  Gain{2,4,11,15} (4 alike) : Gain  Gain=60/(2*pi)
  Gain5 : Gain  Gain=1/car_params.GR
  Gain6 : Gain  Gain=1/car_params.GR
  Gain8 : Gain  Gain=1/10000
  Gain9 : Gain  Gain=3.6
  Mechanical effect : Subsystem
  "Motor Torques " : Scope
  Mux{1,4..5,9..13,20} (9 alike) : Mux  Inputs=2
  Mux{2..3,6..8,14..19,21..24,26..27} (17 alike) : Mux
  Mux25 : Mux  Inputs=3
  Mz_tracking : Scope
  RL : simulink_extras/Transformations/Radians to Degrees
  RL1 : simulink_extras/Transformations/Radians to Degrees
  RR : simulink_extras/Transformations/Radians to Degrees
  RR1 : simulink_extras/Transformations/Radians to Degrees
  Radians to Degrees{,1..2,4,7} (5 alike) : simulink_extras/Transformations/Radians to Degrees
  Radians to Degrees3 : simulink_extras/Transformations/Radians to Degrees  Commented=on
  Rate Transition{,1..5} (6 alike) : RateTransition  OutPortSampleTime=matlab_params.control_system_sample_time
  Rate Transition{6,49..51} (4 alike) : RateTransition  OutPortSampleTimeOpt=Inherit
  Read CM Dict : CarMaker4SL/Read CM Dict  xname=Vhcl.FL.Fx  xsync=off
  Read CM Dict1 : CarMaker4SL/Read CM Dict  xname=Car.LongSlipRL  xsync=off
  Read CM Dict10 : CarMaker4SL/Read CM Dict  xname=Car.vx  xsync=off
  Read CM Dict11 : CarMaker4SL/Read CM Dict  xname=Vhcl.RR.Fz  xsync=off
  Read CM Dict12 : CarMaker4SL/Read CM Dict  xname=Car.Aero.Frc_1.z  xsync=off
  Read CM Dict13 : CarMaker4SL/Read CM Dict  xname=Vhcl.Steer.Ang  xsync=off
  Read CM Dict14 : CarMaker4SL/Read CM Dict  Commented=on  xsync=off
  Read CM Dict15 : CarMaker4SL/Read CM Dict  xname=Car.LongSlipRR  xsync=off
  Read CM Dict16 : CarMaker4SL/Read CM Dict  xname=Car.LongSlipRL  xsync=off
  Read CM Dict17 : CarMaker4SL/Read CM Dict  xname=Car.SlipAngleRR  xsync=off
  Read CM Dict18 : CarMaker4SL/Read CM Dict  xname=Vhcl.FR.Fx  xsync=off
  Read CM Dict19 : CarMaker4SL/Read CM Dict  xname=Vhcl.RR.Fx  xsync=off
  Read CM Dict2 : CarMaker4SL/Read CM Dict  xname=Car.YawRate  xsync=off
  Read CM Dict20 : CarMaker4SL/Read CM Dict  xname=Vhcl.RL.Fx  xsync=off
  Read CM Dict21 : CarMaker4SL/Read CM Dict  xname=Vhcl.FL.Fy  xsync=off
  Read CM Dict22 : CarMaker4SL/Read CM Dict  xname=Vhcl.FR.Fy  xsync=off
  Read CM Dict23 : CarMaker4SL/Read CM Dict  xname=Vhcl.RR.Fy  xsync=off
  Read CM Dict24 : CarMaker4SL/Read CM Dict  xname=Car.WheelSpd_FL  xsync=off
  Read CM Dict25 : CarMaker4SL/Read CM Dict  xname=Car.WheelSpd_FR  xsync=off
  Read CM Dict26 : CarMaker4SL/Read CM Dict  xname=Car.WheelSpd_RL  xsync=off
  Read CM Dict27 : CarMaker4SL/Read CM Dict  xname=Car.WheelSpd_RR  xsync=off
  Read CM Dict28 : CarMaker4SL/Read CM Dict  xname=Vhcl.RL.Fz  xsync=off
  Read CM Dict29 : CarMaker4SL/Read CM Dict  xname=Car.muRoadRL  xsync=off
  Read CM Dict3 : CarMaker4SL/Read CM Dict  xname=Car.CFR.rz  xsync=off
  Read CM Dict30 : CarMaker4SL/Read CM Dict  xname=Car.muRoadRR  xsync=off
  Read CM Dict31 : CarMaker4SL/Read CM Dict  xname=Car.muRoadFL  xsync=off
  Read CM Dict32 : CarMaker4SL/Read CM Dict  xname=Car.muRoadFR  xsync=off
  Read CM Dict33 : CarMaker4SL/Read CM Dict  xname=Car.WFL.Radius  xsync=off
  Read CM Dict34 : CarMaker4SL/Read CM Dict  xname=Car.WFR.Radius  xsync=off
  Read CM Dict35 : CarMaker4SL/Read CM Dict  xname=Car.WRR.Radius  xsync=off
  Read CM Dict36 : CarMaker4SL/Read CM Dict  xname=Car.WRL.Radius  xsync=off
  Read CM Dict37 : CarMaker4SL/Read CM Dict  xname=Car.SlipAngleRL  xsync=off
  Read CM Dict38 : CarMaker4SL/Read CM Dict  xname=Car.SideSlipAngle  xsync=off
  Read CM Dict39 : CarMaker4SL/Read CM Dict  xname=Car.SlipAngleFL  xsync=off
  Read CM Dict4 : CarMaker4SL/Read CM Dict  xname=Car.CFL.rz  xsync=off
  Read CM Dict40 : CarMaker4SL/Read CM Dict  xname=Car.SlipAngleFR  xsync=off
  Read CM Dict41 : CarMaker4SL/Read CM Dict  xname=PT.WFL.Trq_Drive  xsync=off
  Read CM Dict42 : CarMaker4SL/Read CM Dict  xname=PT.WFR.Trq_Drive  xsync=off
  Read CM Dict43 : CarMaker4SL/Read CM Dict  xname=PT.WRL.Trq_Drive  xsync=off
  Read CM Dict44 : CarMaker4SL/Read CM Dict  xname=PT.WRR.Trq_Drive  xsync=off
  Read CM Dict45 : CarMaker4SL/Read CM Dict  xname=Car.SideSlipAngle  xsync=off
  Read CM Dict46 : CarMaker4SL/Read CM Dict  xname=Car.LongSlipFL  xsync=off
  Read CM Dict47 : CarMaker4SL/Read CM Dict  xname=Car.LongSlipFR  xsync=off
  Read CM Dict48 : CarMaker4SL/Read CM Dict  xname=Vhcl.Roll  xsync=off
  Read CM Dict49 : CarMaker4SL/Read CM Dict  xname=Car.Aero.Frc_1.z  xsync=off
  Read CM Dict5 : CarMaker4SL/Read CM Dict  xname=Vhcl.RL.Fy  xsync=off
  Read CM Dict50 : CarMaker4SL/Read CM Dict  xname=Vhcl.YawRate  xsync=off
  Read CM Dict51 : CarMaker4SL/Read CM Dict  xname=Vhcl.YawRate  xsync=off
  Read CM Dict53 : CarMaker4SL/Read CM Dict  xname=Car.Aero.Frc_1.x  xsync=off
  Read CM Dict6 : CarMaker4SL/Read CM Dict  xname=Vhcl.FR.Fz  xsync=off
  Read CM Dict7 : CarMaker4SL/Read CM Dict  xname=Vhcl.FL.Fz  xsync=off
  Read CM Dict8 : CarMaker4SL/Read CM Dict  xname=Car.ax  xsync=off
  Read CM Dict9 : CarMaker4SL/Read CM Dict  xname=Car.ay  xsync=off
  SA calculation : Subsystem
  SA estimate error : Scope  NumInputPorts=4
  SA estimate error1 : Scope  NumInputPorts=4
  SR_i : Scope
  Saturation : Saturate  UpperLimit=50000
  Simulation Results Logging : Subsystem
  Slip angles CM : Scope
  Slip ratios CM1 : Scope
  Slip ratios CM2 : Scope  NumInputPorts=4
  Steering wheel ang-vel2 : CarMaker4SL/Read CM Dict  xname=DM.Steer.AngVel  xsync=off
  Steering wheel ang-vel3 : CarMaker4SL/Read CM Dict  xname=DM.Brake  xsync=off
  Steering wheel angle2 : CarMaker4SL/Read CM Dict  xname=DM.Steer.Ang  xsync=off
  Steering wheel angle3 : CarMaker4SL/Read CM Dict  xname=DM.Gas  xsync=off
  Subsystem : Subsystem
  Subtract : Sum  Inputs=+-
  Subtract1 : Sum  Inputs=+-
  Subtract2 : Sum  Inputs=+-
  Sum : Sum  Inputs=|++
  TV_monitor : Scope  NumInputPorts=9
  TV_monitor1 : Scope  NumInputPorts=5
  "T_requested " : Scope
  To File : ToFile  Filename=MAT_files\MotorRPMS.mat  MatrixName=MotorRpms  SaveFormat=Timeseries
  To File1 : ToFile  Filename=MAT_files\TorqueRequest  MatrixName=TorqueRequest  SaveFormat=Timeseries
  To File10 : ToFile  Filename=analyse_mat/yawRegulator.mat  MatrixName=yaw_reg  SaveFormat=Timeseries
  To File11 : ToFile  Filename=analyse_mat/trueYaw.mat  MatrixName=vhclYaw  SaveFormat=Timeseries
  To File12 : ToFile  Filename=analyse_mat/driverIntentions.mat  MatrixName=driverIntentions  SaveFormat=Timeseries
  To File13 : ToFile  Filename=MAT_files\slip.mat  MatrixName=slipratio  SaveFormat=Timeseries
  To File2 : ToFile  Filename=MAT_files\Speed.mat  MatrixName=VehicleSpeed  SaveFormat=Timeseries
  To File3 : ToFile  Filename=MAT_files\MotorTorques.mat  MatrixName=MotorTorques  SaveFormat=Timeseries
  To File4 : ToFile  Filename=MAT_files\PmPe_FL.mat  MatrixName=PmPe_FL  SaveFormat=Timeseries
  To File5 : ToFile  Filename=MAT_files\PmPe_FR.mat  MatrixName=PmPe_FR  SaveFormat=Timeseries
  To File6 : ToFile  Filename=MAT_files\PmPe_RL.mat  MatrixName=PmPe_RL  SaveFormat=Timeseries
  To File7 : ToFile  Filename=MAT_files\PmPe_RR.mat  MatrixName=PmPe_RR  SaveFormat=Timeseries
  To File8 : ToFile  Filename=MAT_files\SR.mat  MatrixName=SR  SaveFormat=Timeseries
  To File9 : ToFile  Filename=MAT_files\currentDraw.mat  SaveFormat=Timeseries
  Vehicle dynamics analysis JMH : Subsystem  Commented=on
  Vx_kmh : Scope
  "Vx_ms " : Scope
  Yaw rate tracking : Scope
  add_elements : Subsystem
  addall : Subsystem
  addall1 : Subsystem
  ax : Scope
  ay : Scope
  damper force : Scope  NumInputPorts=4
  delta SW : Scope  NumInputPorts=2
  effRadius : Scope
  effectFL_el : Scope
  effectFL_el1 : Scope
  eng rot : Scope
  friction coefficients : Scope
  "longSlip " : Scope
  maxMotorTorques : Scope
  norm_Fx_force : Scope
  rollAngle : Scope
  sideslip angle : Scope
  sideslip angle1 : Scope
  steering angle : Scope
  total z estimated : Scope
  total z force : Scope
  total z force1 : Scope
  total z force2 : Scope  NumInputPorts=4
  whl_speed_cog : Scope
  yawref : Scope  NumInputPorts=2
  wires:
  [T_req] -> To File1/1, "T_requested "/1
  [Mz_error] -> Mux9/1  "error"
  [Mz_ref] -> Mux9/2  "ref"
  Mux9/1 -> Mz_tracking/1
  Mux5/1 -> effectFL_el1/1, To File4/1
  Mux11/1 -> To File5/1
  Mux12/1 -> To File6/1
  Mux13/1 -> To File7/1
  Subsystem/1(Power debug) -> Bus Selector1/1
  Bus Selector1/1 -> Mux5/1  "<Pm_FL>"
  Bus Selector1/2 -> Gain/1, effectFL_el/1, Mux5/2  "<Pe_FL>"
  Bus Selector1/3 -> Mux11/1  "<Pm_FR>"
  Bus Selector1/4 -> Gain12/1, Mux11/2  "<Pe_FR>"
  Bus Selector1/5 -> Mux12/1  "<Pm_RL>"
  Bus Selector1/6 -> Gain13/1, Mux12/2  "<Pe_RL>"
  Bus Selector1/7 -> Mux13/1  "<Pm_RR>"
  Bus Selector1/8 -> Gain14/1, Mux13/2  "<Pe_RR>"
  whl_speed/1 -> Bus Selector2/1
  Bus Selector2/4 -> Mux14/4  "<RR>"
  Bus Selector2/3 -> Mux14/3  "<RL>"
  Bus Selector2/2 -> Mux14/2  "<FR>"
  Bus Selector2/1 -> Mux14/1  "<FL>"
  Mux14/1 -> whl_speed_cog/1
  Fx_est/1 -> Bus Selector3/1
  Bus Selector3/1 -> Mux15/1  "<FL>"
  Bus Selector3/2 -> Mux15/2  "<FR>"
  Bus Selector3/3 -> Mux15/3  "<RL>"
  Bus Selector3/4 -> Mux15/4  "<RR>"
  Mux15/1 -> Fx_estScope/1
  Read CM Dict53/1 -> Aero_Fx/1  "FL"
  Read CM Dict10/1 -> To File2/1, Rate Transition1/1  "V_x"
  Mux10/1 -> "Vx_ms "/1
  Rate Transition1/1 -> Gain9/1, Mux10/1  "V_x"
  Data Type Conversion1/1 -> Mux10/2  "V_est"
  Gain9/1 -> Mux20/1, Vx_kmh/1
  Mux20/1 -> Aero_Fz/1
  Read CM Dict49/1 -> Rate Transition2/1  "FL"
  Rate Transition2/1 -> Mux20/2
  Gain/1 -> Mux21/1  "Current FL"
  Gain12/1 -> Mux21/2  "Current FR"
  Gain13/1 -> Mux21/3  "Current RL"
  Gain14/1 -> Mux21/4  "Current RR"
  Mux21/1 -> To File9/1
  norm_long_tire_force/1 -> Bus Selector5/1
  Bus Selector5/1 -> Mux22/1  "<FL>"
  Bus Selector5/4 -> Mux22/4  "<RR>"
  Bus Selector5/3 -> Mux22/3  "<RL>"
  Bus Selector5/2 -> Mux22/2  "<FR>"
  Mux22/1 -> norm_Fx_force/1
  Rate Transition3/1 -> Discrete Derivative/1
  Saturation/1 -> Fl_derivate/1
  Abs/1 -> Saturation/1
  Discrete Derivative/1 -> Abs/1
  Mux2/1 -> eng rot/1, To File/1
  Read CM Dict27/1 -> Gain3/1
  Read CM Dict26/1 -> Gain1/1
  Gain15/1 -> Mux2/4  "Motor_RPM"
  Gain3/1 -> Gain15/1
  Gain2/1 -> Mux2/3  "Motor_RPM"
  Gain1/1 -> Gain2/1
  Gain11/1 -> Mux2/2  "Motor_RPM"
  Gain10/1 -> Gain11/1
  Read CM Dict25/1 -> Gain10/1
  Read CM Dict24/1 -> Gain7/1
  Gain4/1 -> Mux2/1, Rate Transition3/1  "Motor_RPM"
  Gain7/1 -> Gain4/1
  Radians to Degrees1/1 -> Mux4/2
  Mux4/1 -> steering angle/1
  Read CM Dict3/1 -> Radians to Degrees/1
  Read CM Dict4/1 -> Radians to Degrees1/1
  Radians to Degrees/1 -> Mux4/1
  Read CM Dict48/1 -> Radians to Degrees7/1
  Radians to Degrees7/1 -> rollAngle/1
  Read CM Dict9/1 -> ay/1
  Read CM Dict8/1 -> ax/1
  Read CM Dict1/1 -> "longSlip "/1
  Mux16/1 -> Fx_CM_scope/1
  Read CM Dict18/1 -> Mux16/2  "Fx_FR"
  Read CM Dict19/1 -> Mux16/4  "Fx_RR"
  Read CM Dict20/1 -> Mux16/3  "Fx_RL"
  Read CM Dict/1 -> Mux16/1  "Fx_FL"
  Mux18/1 -> FY_CM/1
  Read CM Dict22/1 -> Mux18/2  "Fy_FR"
  Read CM Dict5/1 -> Mux18/3  "Fy_RL"
  Read CM Dict23/1 -> Mux18/4  "Fy_RR"
  Read CM Dict21/1 -> Mux18/1  "Fy_FL"
  Data Type Conversion10/1 -> Mux3/3  "RL"
  Data Type Conversion7/1 -> Mux3/2  "FR"
  Mux3/1 -> Rate Transition4/1, Fz_CM/1
  Read CM Dict7/1 -> Data Type Conversion8/1
  Read CM Dict11/1 -> Data Type Conversion9/1
  Read CM Dict6/1 -> Data Type Conversion7/1
  Data Type Conversion9/1 -> Mux3/4  "RR"
  Read CM Dict28/1 -> Data Type Conversion10/1
  Data Type Conversion8/1 -> Mux3/1  "FL"
  Read CM Dict30/1 -> Mux6/4  "RR"
  Read CM Dict29/1 -> Mux6/3  "RL"
  Read CM Dict32/1 -> Mux6/2  "FR"
  Mux6/1 -> friction coefficients/1
  Read CM Dict31/1 -> Mux6/1  "FL"
  Gain6/1 -> To File3/1
  Gain5/1 -> "Motor Torques "/1
  Read CM Dict43/1 -> Mux8/3  "Mot_RL"
  Read CM Dict44/1 -> Mux8/4  "Mot_RR"
  Read CM Dict41/1 -> Mux8/1  "Mot_FL"
  Mux8/1 -> Gain6/1, Gain5/1
  Read CM Dict42/1 -> Mux8/2  "Mot_FR"
  Mux17/1 -> effRadius/1
  Data Type Conversion6/1 -> Mux17/4  "R_RR"
  Read CM Dict35/1 -> Data Type Conversion6/1
  Read CM Dict34/1 -> Data Type Conversion13/1
  Data Type Conversion13/1 -> Mux17/2  "R_FR"
  Data Type Conversion11/1 -> Mux17/3  "R_RL"
  Data Type Conversion12/1 -> Mux17/1  "R_FL"
  Read CM Dict36/1 -> Data Type Conversion11/1
  Read CM Dict33/1 -> Data Type Conversion12/1
  Read CM Dict38/1 -> Radians to Degrees2/1
  Radians to Degrees2/1 -> sideslip angle/1
  Mux23/1 -> Extract and scale to deg compare to CM output in individual error/1(SA_CM), Slip angles CM/1
  Read CM Dict40/1 -> FR/1  "FR"
  Read CM Dict39/1 -> FL/1  "FL"
  Read CM Dict17/1 -> RR/1  "RL"
  RR/1 -> Mux23/4
  Read CM Dict37/1 -> RL/1  "RL"
  RL/1 -> Mux23/3
  FR/1 -> Mux23/2
  FL/1 -> Mux23/1
  [yaw_rate_ref] -> Data Type Conversion/1, Simulation Results Logging/1(r_ref)  "r_ref"
  Bus Selector4/4 -> Mux19/4  "<RR>"
  Mux19/1 -> SR_i/1, To File8/1
  Bus Selector4/1 -> Mux19/1  "<FL>"
  Bus Selector4/2 -> Mux19/2  "<FR>"
  Bus Selector4/3 -> Mux19/3  "<RL>"
  "SR "/1 -> Simulation Results Logging/2(SR), Bus Selector4/1
  Data Type Conversion/1 -> Mux1/2  "r_ref"
  Rate Transition/1 -> Mux1/1  "r"
  Mux1/1 -> Yaw rate tracking/1
  Read CM Dict2/1 -> Rate Transition/1  "r"
  Subtract/1 -> Fz_error/1
  Bus Selector6/1 -> Mux7/1  "<Fz_FL>"
  Bus Selector6/2 -> Mux7/2  "<Fz_FR>"
  Bus Selector6/3 -> Mux7/3  "<Fz_RL>"
  Bus Selector6/4 -> Mux7/4  "<Fz_RR>"
  Mux7/1 -> addall1/1(In1), Subtract/1
  Rate Transition4/1 -> Subtract2/2, addall/1(In1), Subtract/2
  addall/1(Out1) -> Subtract1/2, total z force/1
  addall1/1(Out1) -> total z estimated/1, Subtract1/1
  Subtract1/1 -> Fz_error total/1
  Read CM Dict12/1 -> "Aero downforce "/1
  DamperRateLookup/1 -> damper force/1  "Fz_damp_FL"
  Bus Selector7/1 -> DamperRateLookup/1  "<damper_rate_FL>"
  Bus Selector7/2 -> DamperRateLookup1/1  "<damper_rate_FR>"
  Bus Selector7/3 -> DamperRateLookup2/1  "<damper_rate_RL>"
  Bus Selector7/4 -> DamperRateLookup3/1  "<damper_rate_RR>"
  DamperRateLookup1/1 -> damper force/2
  DamperRateLookup2/1 -> damper force/3
  DamperRateLookup3/1 -> damper force/4
  Sensors/1 -> [sensor], Bus Selector8/1, Bus Selector7/1  "V_est"
  Constant/1 -> Fz_error/2
  Bus Selector8/1 -> delta SW/1  "<steering_wheel_angle>"
  Read CM Dict13/1 -> Rate Transition5/1
  Rate Transition5/1 -> Sum/1
  Sum/1 -> delta SW/2
  Constant1/1 -> Sum/2
  [states] -> Bus Selector6/1
  states/1 -> [states]
  SA calculation/1(Out1) -> Extract and scale to deg compare to CM output in individual error/2(In1)
  [sensor] -> SA calculation/1(In1)
  Extract and scale to deg compare to CM output in individual error/1(FL) -> SA estimate error/1
  Extract and scale to deg compare to CM output in individual error/2(FR) -> SA estimate error/2
  Extract and scale to deg compare to CM output in individual error/3(RL) -> SA estimate error/3
  Extract and scale to deg compare to CM output in individual error/4(RR) -> SA estimate error/4
  Radians to Degrees3/1 -> FL steer ang lookup deg/1, FR steer ang lookup deg/1
  Degrees to Radians1/1 -> ?
  FR steer ang lookup deg/1 -> Degrees to Radians1/1
  Degrees to Radians/1 -> ?
  FL steer ang lookup deg/1 -> Degrees to Radians/1
  Bus Selector9/1 -> Radians to Degrees3/1  "<steering_wheel_angle>"
  Read CM Dict45/1 -> Radians to Degrees4/1
  Radians to Degrees4/1 -> sideslip angle1/1
  Mux24/1 -> Extract and scale to deg compare to CM output in individual error1/1(SA_CM), To File13/1, Slip ratios CM1/1
  Read CM Dict47/1 -> FR1/1  "FR"
  Read CM Dict46/1 -> FL1/1  "FL"
  Read CM Dict15/1 -> RR1/1  "RL"
  RR1/1 -> Mux24/4
  Read CM Dict16/1 -> RL1/1  "RL"
  RL1/1 -> Mux24/3
  FR1/1 -> Mux24/2
  FL1/1 -> Mux24/1
  Extract and scale to deg compare to CM output in individual error1/1(FL) -> SA estimate error1/1
  Extract and scale to deg compare to CM output in individual error1/2(FR) -> SA estimate error1/2
  Extract and scale to deg compare to CM output in individual error1/3(RL) -> SA estimate error1/3
  Extract and scale to deg compare to CM output in individual error1/4(RR) -> SA estimate error1/4
  Bus Selector10/1 -> Slip ratios CM2/1, Bus Creator/1  "<SR_FL>"
  Bus Selector10/2 -> Slip ratios CM2/2, Bus Creator/2  "<SR_FR>"
  Bus Selector10/3 -> Slip ratios CM2/3, Bus Creator/3  "<SR_RL>"
  Bus Selector10/4 -> Slip ratios CM2/4, Bus Creator/4  "<SR_RR>"
  [states] -> Bus Selector10/1
  Bus Creator/1 -> Extract and scale to deg compare to CM output in individual error1/2(In1)
  TV_monitoring/1 -> Bus Selector12/1
  Bus Selector12/3 -> TV_monitor/1  "<percentage_delivered_torque>"
  Bus Selector12/4 -> [Mz_error]  "<Mz_error>"
  Bus Selector12/5 -> [yaw_rate_ref]  "<yaw_rate_ref>"
  Bus Selector12/6 -> [T_req]  "<T_req>"
  Bus Selector12/7 -> [Mz_ref]  "<Mz_ref>"
  [Mz_ref] -> TV_monitor1/1, TV_monitor/2
  [yaw_rate_ref] -> TV_monitor/3
  [T_req] -> TV_monitor1/5, TV_monitor/4
  [Mz_error] -> TV_monitor1/2, TV_monitor/5
  Read CM Dict50/1 -> To File11/1
  Rate Transition50/1 -> Mux25/1
  Rate Transition49/1 -> Mux25/2
  Rate Transition51/1 -> Mux25/3
  [yaw_rate_ref] -> Rate Transition50/1
  [Mz_error] -> Rate Transition49/1
  [Mz_ref] -> Rate Transition51/1
  Mux25/1 -> To File10/1
  Steering wheel ang-vel2/1 -> Mux26/2
  Steering wheel angle3/1 -> Mux26/3
  Steering wheel ang-vel3/1 -> Mux26/4
  Steering wheel angle2/1 -> Mux26/1
  Mux26/1 -> total z force1/1, To File12/1
  Bus Selector12/8 -> maxMotorTorques/1, [Max_motor_torque]  "<maxMotorTorque>"
  [Max_motor_torque] -> TV_monitor1/4, TV_monitor/6
  [Max_motor_torque] -> add_elements/1(In1)
  add_elements/1(Out1) -> TV_monitor/7
  ? -> Bus Selector11/1
  [states] -> Bus Selector/1
  Bus Selector/1 -> Gain8/1  "<power>"
  Bus Selector/2 -> total z force2/2  "<Input_throttle>"
  Bus Selector/3 -> total z force2/3  "<Input_brake>"
  Bus Selector/4 -> total z force2/4  "<KERS_pos>"
  Gain8/1 -> total z force2/1
  Read CM Dict51/1 -> yawref/1
  [yaw_rate_ref] -> Rate Transition6/1
  Rate Transition6/1 -> yawref/2
  Constant2/1 -> Fz_acc_error/2
  Subtract2/1 -> Fz_acc_error/1
  Bus Selector13/1 -> Mux27/1  "<FL>"
  Bus Selector13/2 -> Mux27/2  "<FR>"
  Bus Selector13/3 -> Mux27/3  "<RL>"
  Bus Selector13/4 -> Mux27/4  "<RR>"
  Fz_acc/1 -> Bus Selector13/1
  Mux27/1 -> Subtract2/1
